simulink model "nivel1"  (R2020b)
settings: Solver=VariableStepAuto  StartTime=0.0  StopTime=10.0  RelTol=1e-3
settings Model: Creator=GoniR  LastModifiedBy=GoniR
settings ConfigComp: PLC_TargetIDE=codesys23

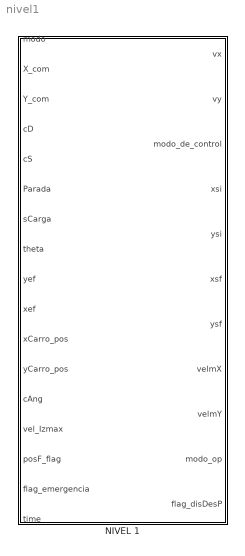
== system nivel1 ==
  NIVEL 1 : Stateflow chart  TreatAsAtomicUnit=on
      settings: PortSchema="{\"entries\":[{\"content\":{\"sides\":[{\"content\":{\"connectorIds\":[\"In13\",\"In1\",\"In2\",\"In5\",\"In6\",\"In10\",\"In7\",\"In14\",\"In3\",\"In4\",\"In9\",\"In12\",\"In8\",\"In15\",\"In17\",\"In16\",\"In11\"]},\"type\":\"ConnectorPlacement.EquallySpacedRectSide\",\"uuid\":\"1e4dd542-1771-4859-b91f-fc1cb250280a\"},{\"content\":{\"connectorIds\":[\"Out1\",\"Out2\",\"Out9\",\"Out7\",\"Out6\",\"Out8\",\"Out5\",\"Out4\",\"Out3\",\"Out10\",\"Out11\"],\"side\":\"RIGHT\"},\"type\":\"ConnectorPlacement.EquallySpacedRectSide\",\"uuid\":\"bb5e6521-c449-4a1c-9147-094c14f63665\"},{\"content\":{\"connectorIds\":[],\"side\":\"TOP\"},\"type\":\"ConnectorPlacement.EquallySpacedRectSide\",\"uuid\":\"54352a45-add1-4eb7-bb1e-2f57d731739f\"},{\"content\":{\"connectorIds\":[],\"side\":\"HIDDEN\"},\"type\":\"ConnectorPlacement.EquallySpacedRectSide\",\"uuid\":\"3e291a91-093a-4ab5-80ab-be4d5a353953\"}]},\"type\":\"ConnectorPlacement.EquallySpacedConnector\",\"uuid\":\"db8c49e8-a9b8-459f-b7fa-0d865c8e3061\"}],\"packageUris\":[\"http://schema.mathworks.com/mf0/Connector/R2020b\"],\"version\":\"1.0\"}"

== stateflow chart nivel1/NIVEL 1 ==
  state Nivel1
    state Spreder [parallel]
      settings: executionOrder=1
      state Descargado
        en:
        Scargado=0
      state Cargado
        en:
        Scargado=1
      (default) -> Descargado
      Descargado -> Cargado : [sCarga==1]
      Cargado -> Descargado : [sCarga==0]
    state controlAngulo [parallel]
      settings: executionOrder=2
      state Desactivado
      state Activado
      (default) -> Activado
      Activado -> Desactivado : [cAng==0]
      Desactivado -> Activado : [cAng==1]
    state modoOperacion [parallel]
      settings: executionOrder=3
      state Automatico
        state CicloSimple
          state descaragBarco
            en :
            xsi=xCarro_pos;
            ysi=yCarro_pos;
            xsf=xef;
            ysf=yef;
            velmX=4;
            velmY=vel_Izmax
            modo_de_control=1
            du:
            error=Calc_error(xsf,xCarro_pos,ysf,yCarro_pos);
          state cargaBarco
            en :
            xsi=xCarro_pos;
            ysi=yCarro_pos;
            xsf=xef;
            ysf=yef;
            velmX=4;
            velmY=vel_Izmax;
            modo_de_control=1;
            du:
            error=Calc_error(xsf,xCarro_pos,ysf,yCarro_pos);
          state standby
            en :
            modo_op = 2;
          state idaBarco
            en :
            xsi=xCarro_pos;
            ysi=yCarro_pos;
            xsf=xef;
            ysf=yef;
            velmX=4;
            velmY=vel_Izmax;
            modo_de_control=1;
            du:
            error=Calc_error(xsf,xCarro_pos,ysf,yCarro_pos);
          state vueltaMuelle
            en :
            xsi=xCarro_pos
            ysi=yCarro_pos
            xsf=xef
            ysf=yef
            velmX=4
            velmY=vel_Izmax
            modo_de_control=1
            du:
            error=Calc_error(xsf,xCarro_pos,ysf,yCarro_pos);
          Nivel1.modoOperacion.Automatico.CicloSimple.standby -> Nivel1.modoOperacion.Automatico.CicloSimple.cargaBarco [order 1] : [Scargado==1 && xCarro_pos<30 ]
          Nivel1.modoOperacion.Automatico.CicloSimple.standby -> Nivel1.modoOperacion.Automatico.CicloSimple.descaragBarco [order 2] : [Scargado==1 && xCarro_pos>30]
          (default) -> Nivel1.modoOperacion.Automatico.CicloSimple.standby
          Nivel1.modoOperacion.Automatico.CicloSimple.standby -> vueltaMuelle [order 3] : [Scargado==0 && xCarro_pos>30]
          Nivel1.modoOperacion.Automatico.CicloSimple.standby -> idaBarco [order 4] : [Scargado==0 && xCarro_pos<30]
        state standby
          en:
          error=inf;
          modo_op = 1;
        state CicloDoble
          state cargaBarco
            en :
            xsi=xCarro_pos;
            ysi=yCarro_pos;
            xsf=xef;
            ysf=yef;
            velmX=4;
            velmY=vel_Izmax;
            error=inf;
            modo_de_control=1;
            flagD_cB=1;
            du :
            error=Calc_error(xsf,xCarro_pos,ysf,yCarro_pos);
          state standby
            en:
            modo_op = 3;
            flagcD=1;
            cont=cont+1;
            if(cont==2)
            flagcD=0;
            cont=0;
            end
          state descaragBarco
            en :
            xsi=xCarro_pos;
            ysi=yCarro_pos;
            xsf=xef;
            ysf=yef;
            velmX=4;
            velmY=vel_Izmax;
            error=inf;
            modo_de_control=1;
            flagD_cB=0;
            du:
            error=Calc_error(xsf,xCarro_pos,ysf,yCarro_pos);
          Nivel1.modoOperacion.Automatico.CicloDoble.standby -> Nivel1.modoOperacion.Automatico.CicloDoble.cargaBarco [order 1] : [xCarro_pos<30]
          (default) -> Nivel1.modoOperacion.Automatico.CicloDoble.standby
          Nivel1.modoOperacion.Automatico.CicloDoble.standby -> Nivel1.modoOperacion.Automatico.CicloDoble.descaragBarco [order 2] : [xCarro_pos>30]
        Nivel1.modoOperacion.Automatico.standby -> CicloSimple [order 1] : [cS==115 && posF_flag]
        CicloSimple -> Nivel1.modoOperacion.Automatico.standby : [Parada==112 ]
        (default) -> Nivel1.modoOperacion.Automatico.standby
        Nivel1.modoOperacion.Automatico.standby -> CicloDoble [order 2] : [(cD==100 && posF_flag)|| flagcD]
        CicloDoble -> Nivel1.modoOperacion.Automatico.standby : [Parada==112 ]
      state modoManual
        en :
        modo_op = 0;
        xsi=xCarro_pos;
        ysi=yCarro_pos;
        vx=0;
        vy=0;
        time_a=time;
        vx_a=0;
        vy_a=0;
        error=0;
        delta_t=0;
        modo_de_control=0;
        dist_desp=yCarro_pos-20;
        if(dist_desp>2)
        flag_disDesP=1;
        else
        flag_disDesP=0;
        end
        du :
        delta_t=time-time_a;
        [vx,vy]=Calc_v(delta_t,vx_a,vy_a,X_com,Y_com);
        time_a=time;
        vx_a=vx;
        vy_a=vy;
      state transicion
        en:
        time_a=time;
        delta_t=0;
        du:
        delta_t=time-time_a;
        [vx,vy]=Calc_v1(delta_t,vx,vy);
        time_a=time;
        ex:
        vx = 0;
        vy = 0;
      state transicion1
        en:
        time_a=time
        delta_t=0
        du:
        delta_t=time-time_a;
        [vx,vy]=Calc_v1(delta_t,vx,vy);
        time_a=time;
        ex:
        vx = 0
        vy = 0
      (default) -> modoManual
      transicion -> Automatico : [abs(vx)<0.1 && abs(vy)<0.01]
      modoManual -> transicion : [modo==97 && (dist_desp>2 || xCarro_pos>30)   ]
      Automatico -> transicion1 [order 1] : [error<2 && theta <0.05 || modo==109]
      transicion1 -> modoManual : [abs(vx)<0.1 && abs(vy)<0.01]
      Automatico -> transicion1 [order 2] : [flag_emergencia]
  (default) -> Nivel1
  data: delta_t2 function_input double; vx_a2 function_input double; vy_a2 function_input double; vx2 function_output; vy2 function_output; er function_output; xf function_input; xpos function_input; yf function_input; ypos function_input; delta_t1 function_input double; vx_a1 function_input double; vy_a1 function_input double; vx1 function_output; vy1 function_output; X_com1 function_input; Y_com1 function_input; X_com input; Y_com input; vx output; opManual local; vy output; yef input; xef input; velmY output; velmX output; ysf output; ysi output; xsi output; xsf output; cD input; Scargado local; cS input; sCarga input; cAng input; xCarro_pos input; Parada input; time input; time_i local; vx_a local; time_a local; yCarro_pos input; error local; vy_a local; delta_t local; modo input; modo_de_control output; flagD_cB local; cont local =0; theta input; dist_desp local; modo_op output; vel_Izmax input; flag_emergencia input; posF_flag input; flag_disDesP output; flagcD local =0
  function [vx2,vy2]=Calc_v1(delta_t2,vx_a2,vy_a2):
    | function [vx2,vy2]=Calc_v1(delta_t2,vx_a2,vy_a2)
    | if (vx_a2 < 0 )
    |     vx2=0.2*(delta_t2)+vx_a2;
    | else
    |     vx2=-0.2*(delta_t2)+vx_a2;
    | end
    | if (vy_a2 < 0)
    |     vy2=0.2*(delta_t2)+vy_a2;
    | else
    |     vy2=-0.2*(delta_t2)+vy_a2;
    | end
    | end
  function er=Calc_error(xf,xpos,yf,ypos):
    | function er=Calc_error(xf,xpos,yf,ypos)
    |     er=((xf-xpos)^2+(yf-ypos)^2)^0.5;
  function [vx1,vy1]=Calc_v(delta_t1,vx_a1,vy_a1,X_com1,Y_com1):
    | function [vx1,vy1]=Calc_v(delta_t1,vx_a1,vy_a1,X_com1,Y_com1)
    | if (X_com1 == 29 && vx_a1<4)
    |     vx1=0.8*(delta_t1)+vx_a1;
    | elseif (X_com1 == 28 && vx_a1 > -4 )
    |     vx1=-0.8*(delta_t1)+vx_a1;
    | else
    |     vx1=vx_a1;
    | end
    | if (Y_com1 == 31 && vy_a1<1.5)
    |     vy1=0.8*(delta_t1)+vy_a1;
    | elseif (Y_com1==30 && vy_a1>-1.5)
    |     vy1=-0.8*(delta_t1)+vy_a1;
    | else
    |     vy1=vy_a1;
    | end
    | 
    | end
